simulink model "Node"  (R2021b)
settings: Solver=VariableStepAuto  StartTime=0.0  StopTime=10.0  RelTol=1e-3
settings Model: Creator=Rob  LastModifiedBy=Rob
settings DataIOCC: ExternalInput=[t, u,zeta,tau,past,prevsus]  LoadExternalInput=on

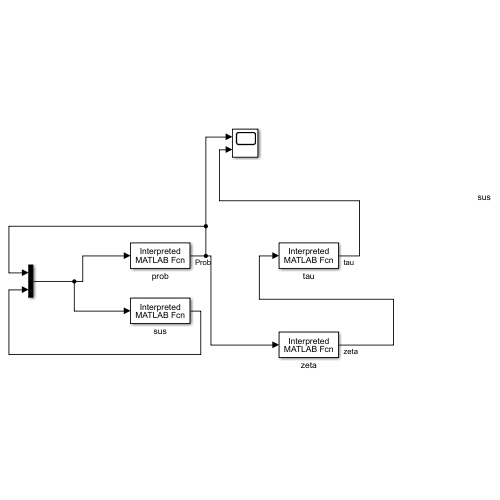
[thumbnail: Simulink's stored preview of the top-level diagram]
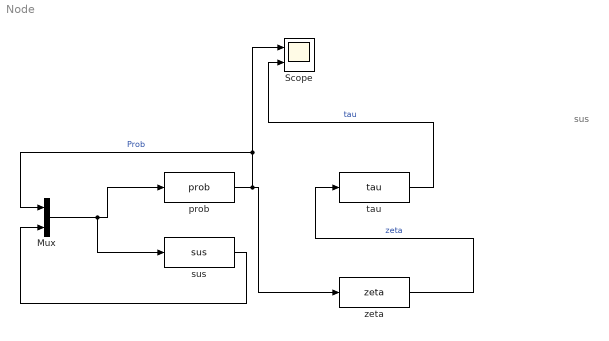
== system Node ==
  note: sus
  Mux : Mux  Inputs=2
  Scope : Scope  NumInputPorts=2
  prob : MATLABFcn  MATLABFcn=prob  OutputDimensions=2  Output1D=off
  sus : MATLABFcn  MATLABFcn=sus  OutputDimensions=2
  tau : MATLABFcn  MATLABFcn=tau  OutputDimensions=2
  zeta : MATLABFcn  MATLABFcn=zeta  OutputDimensions=2
  wires:
  Mux/1 -> sus/1, prob/1
  sus/1 -> Mux/2
  prob/1 -> zeta/1, Scope/1, Mux/1  "Prob"
  zeta/1 -> tau/1  "zeta"
  tau/1 -> Scope/2  "tau"
